simulink model "UpDownPendulumMOD22"  (R2025b)
settings: Solver=ode1  StartTime=0.0  StopTime=200  FixedStep=0.001  RelTol=1e-3
undefined symbols (not defined in the file): magnitude
libraries: simulink x6, slpidlib x5, raspberrypiCommlib x2, raspberrypiBasiclib x1
(part 2 of 2)

== system UpDownPendulumMOD22/Swing up and stabilization control/Swing up control + position control/Voltage sign switching depending on pendulum position ==
  angular velocity : Inport
  control voltage : Inport  Port=2
  upper / lower zone detection : Inport  Port=3
  Enable : EnablePort
  Gain : Gain  Gain=-1
  Gain2 : Gain  Gain=-1
  upper or lower : Switch  Criteria=u2 > Threshold  Threshold=0.5  SaturateOnIntegerOverflow=off  InputSameDT=off
  zero velocity : Switch  SaturateOnIntegerOverflow=off  InputSameDT=off
  control voltage to the motor : Outport
  wires:
  Gain/1 -> upper or lower/3
  zero velocity/1 -> upper or lower/1, Gain/1
  control voltage/1 -> zero velocity/1, Gain2/1
  Gain2/1 -> zero velocity/3
  angular velocity/1 -> zero velocity/2
  upper or lower/1 -> control voltage to the motor/1
  upper / lower zone detection/1 -> upper or lower/2

== system UpDownPendulumMOD22/Swing up and stabilization control/Swing up control + position control/first move ==
  pulse : Inport
  Add1 : Sum  Inputs=+-
  Product : Product  RndMeth=Zero
  control v2 : Constant  Value=0.4
  initialization : Outport
  wires:
  control v2/1 -> Add1/1, Product/1
  Product/1 -> Add1/2
  pulse/1 -> Product/2
  Add1/1 -> initialization/1

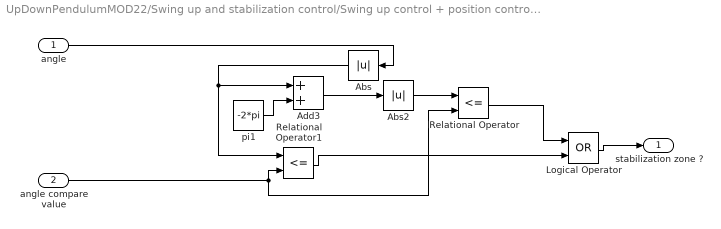
== system UpDownPendulumMOD22/Swing up and stabilization control/Swing up control + position control/stabilization zone detection  ==
  angle : Inport
  angle compare value : Inport  Port=2
  Abs : Abs  SaturateOnIntegerOverflow=off
  Abs2 : Abs  SaturateOnIntegerOverflow=off
  Add3 : Sum
  Logical Operator : Logic  Operator=OR  AllPortsSameDT=off  OutDataTypeStr=boolean
  Relational Operator : RelationalOperator  Operator=<=  OutDataTypeStr=boolean  InputSameDT=off
  Relational Operator1 : RelationalOperator  Operator=<=  OutDataTypeStr=boolean  InputSameDT=off
  pi1 : Constant  Value=-2*pi
  stabilization zone ? : Outport
  wires:
  Abs/1 -> Add3/1, Relational Operator1/1
  Relational Operator1/1 -> Logical Operator/2
  pi1/1 -> Add3/2
  Add3/1 -> Abs2/1
  Relational Operator/1 -> Logical Operator/1
  Abs2/1 -> Relational Operator/1
  angle/1 -> Abs/1
  Logical Operator/1 -> stabilization zone ?/1
  angle compare value/1 -> Relational Operator1/2, Relational Operator/2

== system UpDownPendulumMOD22/Swing up and stabilization control/Swing up control + position control/Extra PI control for cart position/PID Controller with D part filter1 ==
  In_1 : Inport
  D : Gain  Gain=D  SaturateOnIntegerOverflow=on  OutDataTypeStr=Inherit: Same as input  ParamDataTypeStr=Inherit: Same as input
  Derivative : Derivative
  Integral : TransferFcn  Numerator=[I]  Denominator=[1 0]
  Pendulum Velocity  Filter : TransferFcn  Numerator=[1e4]  Denominator=[1 70.7 1e4]
  Proportional : Gain  Gain=P  SaturateOnIntegerOverflow=on  OutDataTypeStr=Inherit: Same as input  ParamDataTypeStr=Inherit: Same as input
  Sum : Sum  Inputs=+++  InputSameDT=on  SaturateOnIntegerOverflow=on  OutDataTypeStr=Inherit: Same as first input
  Out_1 : Outport  InitialOutput=0
  wires:
  Proportional/1 -> Sum/1
  Integral/1 -> Sum/2
  Derivative/1 -> Pendulum Velocity  Filter/1
  In_1/1 -> Integral/1, Proportional/1, D/1
  Sum/1 -> Out_1/1
  D/1 -> Derivative/1
  Pendulum Velocity  Filter/1 -> Sum/3

== matlab function UpDownPendulumMOD22/Cart Position_Pendulum Angle1/Encoder_data/MATLAB Function ==
  data: data input uint8 size=[1 12]; motor output; pendulum output; flags output; valid output
function [motor, pendulum, flags, valid] = unpack_spi(data)

% Checksum
chk = uint8(0);
for i = 1:9
    chk = bitxor(chk, data(i));
end
valid = logical(chk == data(10));

% Motor — bytes 1-4 little-endian
motor_int = int32(data(1)) + ...
        bitshift(int32(data(2)), 8) + ...
        bitshift(int32(data(3)), 16) + ...
        bitshift(int32(data(4)), 24);

% Pendulum — bytes 5-8 little-endian
pend_int = int32(data(5)) + ...
           bitshift(int32(data(6)), 8) + ...
           bitshift(int32(data(7)), 16) + ...
           bitshift(int32(data(8)), 24);

% Flags
flags = uint8(data(9));

% Output as single (32-bit float) for use in control blocks
motor    = double(motor_int);
pendulum = single(pend_int);

end

== matlab function UpDownPendulumMOD22/Feedback DAC1/MATLAB Function ==
  data: v_desired input; bytes output; v_ref input
function bytes = voltToMCP4725(v_desired, v_ref)
    % v_desired: desired output voltage (0 to v_ref)
    % v_ref: DAC supply voltage (5.0)
    dacVal = uint16(round((v_desired / v_ref) * 4095));
    dacVal = min(dacVal, uint16(4095));
    b0 = uint8(64);                        % 0x40 command byte
    b1 = uint8(bitshift(dacVal, -4));      % upper 8 bits
    b2 = uint8(bitshift(bitand(dacVal, uint16(15)), 4)); % lower 4 bits
    bytes = [b0; b1; b2];
end

== matlab function UpDownPendulumMOD22/Cart Position_Pendulum Angle1/DO Generate ==
  data: D1 output; t input
%%pendulum 10
function D1  = generate_DO(t)
    if t <= 0.002
        D1 = 1;  % RESET on first sample
    else
        D1 = 0;
    end
end



%%pendulum 5
% function [D1, D2] = generate_DO(counter, t)
%     if t <= 0.002
%         D1 = 1;  % RESET on first sample
%         % D2 = 0;
%     else
%         D1 = 0;
%     %     D2 = 0;
%         % if mod(counter, 4) < 2
%         %     D1 = 0;
%         %     D2 = 0;
%         % else
%         %     D1 = 1;
%         %     D2 = 0;
%         % end
%     end
% end


%%pendulum 4
% function DO = generate_DO(counter)
%     switch counter
%         case 0
%             DO = 4;  % Reset/idle
%         case 1
%             DO = 1;  % Set DO=1 (ESP32 prepares high byte)
%         case 2
%             DO = 4;  % Keep DO=1 (Simulink reads high byte)        
%         case 3
%             DO = 4;  % Keep DO=1 (Simulink reads high byte)        
%         case 4
%             DO = 2;  % Keep DO=1 (Simulink reads high byte)        
% %         case 3
% %             DO = 1;  % Keep DO=1 (Simulink reads high byte)
% %         case 3
% %             DO = 2; %seperations
% %         case 5
% %             DO = 4; %seperations
% %         case 4
% %             DO = 2;  % Set DO=2 (ESP32 prepares low byte)
% %         case 7
% %             DO = 2;  % Keep DO=2 (Simulink reads low byte)
% %         case 8
% %             DO = 2;  % Keep DO=2 (Simulink reads low byte)
% %         case 9
% %             DO = 4;  % Unlatch
%         otherwise
%             DO = 4;
%     end
% end
% 
% function DO = generate_DO(counter)
%     % Just toggle between 0 and 1
%     if counter == 0
%         DO = 1;  % Motor state
%     else
%         DO = 0;  % Pendulum state
%     end
% end
